simulink model "hyd_hyb_2_int_cont_Final"  (Simulink 8.2)
settings: Solver=ode4  StartTime=0  StopTime=3005  FixedStep=0.01  MaxStep=.4  RelTol=1e-8
InitFcn:
  | const_3_new
values from neighbouring files (symbols this model uses):
  Af = 6.3    [brk_enrg.m]    (also in brk_enrg_1.m)
  BSFC_906_205 = [3.5684 4.3466 5.1668 6.0769 6.988 7.8992 8.8104 9.7336 10.8548 11.9809 13.1112 14.2571 ... (663 elements, 39x17)]    [BSFC_map_906_205.mat]
  Cd = 0.55    [brk_enrg.m]    (also in brk_enrg_1.m)
  den = 1.202    [brk_enrg.m]    (also in brk_enrg_1.m)
  fr = 0.01    [brk_enrg.m]    (also in brk_enrg_1.m)
undefined symbols (not defined in the file or in its folder): clutchRise, down_spd_2, down_spd_3, down_spd_4, down_spd_c, Driving_Cycle, fuel_density, gearshift, I_wheel, Idle_spd_eng_906, M1_hydr, p_v_15, pmax_125, qv_125, Rw, sec_eng_sfc_map, T0, T1, T_max_906, T_min, TC_spd_ratio_max, teta_new_10, torque_convertor, Twait, up_spd_1, up_spd_2, up_spd_3, up_spd_c, v_p_10, v_p_15, v_p_5
libraries: neural x1742, fl_lib x43, nesl_utility x30, sdl_lib x14, simulink x4, simulink_need_slupdate x1
(part 4 of 26)

== system hyd_hyb_2_int_cont_Final/controller1/optimized controller/SOC under 0.5/col_e_f/net_col_e_f_2_4/Layer 1 ==
  "p{1}" : Inport  PortDimensions=2
  Delays 1 : Subsystem
  "IW{1,1}" : Subsystem
  "b{1}" : Constant  Value=[3.1870017165883615;1.5888517108202425;-0.37804805527583374;-1.1180149001441948;-3.2150121471194906]
  netsum : Sum  Inputs=2  SaturateOnIntegerOverflow=on  InputSameDT=on  OutDataTypeStr=Inherit: Same as first input
  tansig : neural/Transfer Functions/tansig
  "a{1}" : Outport  InitialOutput=[0;0;0;0;0]
  wires:
  "p{1}"/1 -> Delays 1/1("p{1}")
  Delays 1/1("pd{1,1}") -> "IW{1,1}"/1("pd{1,1}")
  "IW{1,1}"/1("iz{1,1}") -> netsum/1
  "b{1}"/1 -> netsum/2
  netsum/1 -> tansig/1
  tansig/1 -> "a{1}"/1

== system hyd_hyb_2_int_cont_Final/controller1/optimized controller/SOC under 0.5/col_e_f/net_col_e_f_2_4/Layer 2 ==
  "a{1} " : Inport  PortDimensions=5
  Delays 1 : Subsystem
  "LW{2,1}" : Subsystem
  "b{2}" : Constant  Value=[-2.1782011876605245;2.0554076448718699;1.2298603286219902;-0.89936716113614468;-0.28721557149157961;-0.24676230996003104;-0.6440977364861179;-1.2306338127509255;1.7211311759643211;-2.0651300272875792]
  netsum : Sum  Inputs=2  SaturateOnIntegerOverflow=on  InputSameDT=on  OutDataTypeStr=Inherit: Same as first input
  tansig : neural/Transfer Functions/tansig
  "a{2}" : Outport  InitialOutput=[0;0;0;0;0;0;0;0;0;0]
  wires:
  "a{1} "/1 -> Delays 1/1("p{2}")
  Delays 1/1("pd{2,1}") -> "LW{2,1}"/1("ad{2,1}")
  "LW{2,1}"/1("lz{2,1}") -> netsum/1
  "b{2}"/1 -> netsum/2
  netsum/1 -> tansig/1
  tansig/1 -> "a{2}"/1

== system hyd_hyb_2_int_cont_Final/controller1/optimized controller/SOC under 0.5/col_e_f/net_col_e_f_2_4/Layer 3 ==
  "a{2} " : Inport  PortDimensions=10
  Delays 1 : Subsystem
  "LW{3,2}" : Subsystem
  "b{3}" : Constant  Value=0.88069891967558567
  netsum : Sum  Inputs=2  SaturateOnIntegerOverflow=on  InputSameDT=on  OutDataTypeStr=Inherit: Same as first input
  purelin : neural/Transfer Functions/purelin
  "a{3}" : Outport  InitialOutput=0
  wires:
  "a{2} "/1 -> Delays 1/1("p{3}")
  Delays 1/1("pd{3,2}") -> "LW{3,2}"/1("ad{3,2}")
  "LW{3,2}"/1("lz{3,2}") -> netsum/1
  "b{3}"/1 -> netsum/2
  netsum/1 -> purelin/1
  purelin/1 -> "a{3}"/1

== system hyd_hyb_2_int_cont_Final/controller1/optimized controller/SOC under 0.5/col_e_f/net_col_e_f_2_4/Process Input 1 ==
  x : Inport  PortDimensions=2
  fixunknowns : neural/Processing Functions/fixunknowns  inputSize=2  indices=[1 2]
  mapminmax : neural/Processing Functions/mapminmax  xmin=[0.0064010483261946602;0.40225]  xmax=[1.009090909090909;0.527752]  ymin=-1  ymax=1
  removeconstantrows : neural/Processing Functions/removeconstantrows  inputSize=2  keep=[1 2]
  p : Outport  PortDimensions=2
  wires:
  x/1 -> fixunknowns/1
  fixunknowns/1 -> removeconstantrows/1
  removeconstantrows/1 -> mapminmax/1
  mapminmax/1 -> p/1

== system hyd_hyb_2_int_cont_Final/controller1/optimized controller/SOC under 0.5/col_e_f/net_col_e_f_2_4/Process Output 1 ==
  a : Inport  PortDimensions=1
  mapminmax_reverse : neural/Processing Functions/mapminmax_reverse  xmin=0  xmax=0.96424337740449761  ymin=-1  ymax=1
  removeconstantrows_reverse : neural/Processing Functions/removeconstantrows_reverse  inputSize=1  constants=zeros(0,1)  rearrange=1
  y : Outport  PortDimensions=1
  wires:
  a/1 -> mapminmax_reverse/1
  mapminmax_reverse/1 -> removeconstantrows_reverse/1
  removeconstantrows_reverse/1 -> y/1

== system hyd_hyb_2_int_cont_Final/controller1/optimized controller/SOC under 0.5/col_e_f/net_col_e_f_4_5/Layer 1 ==
  "p{1}" : Inport  PortDimensions=2
  Delays 1 : Subsystem
  "IW{1,1}" : Subsystem
  "b{1}" : Constant  Value=[6.2806292292580581;5.6430633337179623;4.9428699040675612;-4.2619922724486017;-3.6535514778845468;2.9896328681278797;2.3029778837955286;1.6337499102133759;-0.88051813078209484;0.2793526252740125;0.50789388949179792;-1.0078514961654155;1.4630287312614616;2.3246897312524242;2.9777230797325829;-3.5795229522621734;4.2851583321352358;-4.986226223743337;-5.6313909550551342;6.2616529893046176]
  netsum : Sum  Inputs=2  SaturateOnIntegerOverflow=on  InputSameDT=on  OutDataTypeStr=Inherit: Same as first input
  tansig : neural/Transfer Functions/tansig
  "a{1}" : Outport  InitialOutput=[0;0;0;0;0;0;0;0;0;0;0;0;0;0;0;0;0;0;0;0]
  wires:
  "p{1}"/1 -> Delays 1/1("p{1}")
  Delays 1/1("pd{1,1}") -> "IW{1,1}"/1("pd{1,1}")
  "IW{1,1}"/1("iz{1,1}") -> netsum/1
  "b{1}"/1 -> netsum/2
  netsum/1 -> tansig/1
  tansig/1 -> "a{1}"/1

== system hyd_hyb_2_int_cont_Final/controller1/optimized controller/SOC under 0.5/col_e_f/net_col_e_f_4_5/Layer 2 ==
  "a{1} " : Inport  PortDimensions=20
  Delays 1 : Subsystem
  "LW{2,1}" : Subsystem
  "b{2}" : Constant  Value=[1.6889050227737452;-1.5966398366125047;-1.5114553194028437;-1.4193609656938586;-1.3563280059510718;1.2527618415722073;1.1049860773470304;1.193805294938213;1.0220627774516799;-0.89895684788464469;-0.82709085724455877;0.78466162175281673;0.63003503504393021;0.56915459741996099;-0.45812028507076141;0.39250587067480053;0.3072138621800331;-0.20098633077147457;0.049397562122670803;0.036839924743362153;-0.03660385580770284;-0.14959783393044784;0.20236800626272414;0.29924031316589073;-0.37480244151300107;0.51487980632788588;0.56519308531635493;-0.6582920010771226;0.72211111302575659;-0.82064724071454276;0.90350102117262521;-0.96842037466691033;-1.1096684688881748;1.1383114710157722;-1.2625762588771776;-1.3484015255301616;-1.5727816552062366;1.4561588594730721;-1.6262096633611691;-1.7069579131524728]
  netsum : Sum  Inputs=2  SaturateOnIntegerOverflow=on  InputSameDT=on  OutDataTypeStr=Inherit: Same as first input
  tansig : neural/Transfer Functions/tansig
  "a{2}" : Outport  InitialOutput=[0;0;0;0;0;0;0;0;0;0;0;0;0;0;0;0;0;0;0;0;0;0;0;0;0;0;0;0;0;0;0;0;0;0;0;0;0;0;0;0]
  wires:
  "a{1} "/1 -> Delays 1/1("p{2}")
  Delays 1/1("pd{2,1}") -> "LW{2,1}"/1("ad{2,1}")
  "LW{2,1}"/1("lz{2,1}") -> netsum/1
  "b{2}"/1 -> netsum/2
  netsum/1 -> tansig/1
  tansig/1 -> "a{2}"/1

== system hyd_hyb_2_int_cont_Final/controller1/optimized controller/SOC under 0.5/col_e_f/net_col_e_f_4_5/Layer 3 ==
  "a{2} " : Inport  PortDimensions=40
  Delays 1 : Subsystem
  "LW{3,2}" : Subsystem
  "b{3}" : Constant  Value=0.083693897910831885
  netsum : Sum  Inputs=2  SaturateOnIntegerOverflow=on  InputSameDT=on  OutDataTypeStr=Inherit: Same as first input
  purelin : neural/Transfer Functions/purelin
  "a{3}" : Outport  InitialOutput=0
  wires:
  "a{2} "/1 -> Delays 1/1("p{3}")
  Delays 1/1("pd{3,2}") -> "LW{3,2}"/1("ad{3,2}")
  "LW{3,2}"/1("lz{3,2}") -> netsum/1
  "b{3}"/1 -> netsum/2
  netsum/1 -> purelin/1
  purelin/1 -> "a{3}"/1

== system hyd_hyb_2_int_cont_Final/controller1/optimized controller/SOC under 0.5/col_e_f/net_col_e_f_4_5/Process Input 1 ==
  x : Inport  PortDimensions=2
  fixunknowns : neural/Processing Functions/fixunknowns  inputSize=2  indices=[1 2]
  mapminmax : neural/Processing Functions/mapminmax  xmin=[0.012323778098949922;0.30892799999999998]  xmax=[1.009090909090909;0.60337499999999999]  ymin=-1  ymax=1
  removeconstantrows : neural/Processing Functions/removeconstantrows  inputSize=2  keep=[1 2]
  p : Outport  PortDimensions=2
  wires:
  x/1 -> fixunknowns/1
  fixunknowns/1 -> removeconstantrows/1
  removeconstantrows/1 -> mapminmax/1
  mapminmax/1 -> p/1

== system hyd_hyb_2_int_cont_Final/controller1/optimized controller/SOC under 0.5/col_e_f/net_col_e_f_4_5/Process Output 1 ==
  a : Inport  PortDimensions=1
  mapminmax_reverse : neural/Processing Functions/mapminmax_reverse  xmin=0  xmax=1  ymin=-1  ymax=1
  removeconstantrows_reverse : neural/Processing Functions/removeconstantrows_reverse  inputSize=1  constants=zeros(0,1)  rearrange=1
  y : Outport  PortDimensions=1
  wires:
  a/1 -> mapminmax_reverse/1
  mapminmax_reverse/1 -> removeconstantrows_reverse/1
  removeconstantrows_reverse/1 -> y/1

== system hyd_hyb_2_int_cont_Final/controller1/optimized controller/SOC under 0.5/net_loc_rod_2_5/Layer 1/Delays 1 ==
  "p{1}" : Inport  PortDimensions=2
  mux : Mux  Inputs=1
  "pd{1,1}" : Outport
  wires:
  "p{1}"/1 -> mux/1
  mux/1 -> "pd{1,1}"/1

== system hyd_hyb_2_int_cont_Final/controller1/optimized controller/SOC under 0.5/net_loc_rod_2_5/Layer 1/IW{1,1} ==
  "pd{1,1}" : Inport  PortDimensions=2
  "IW{1,1}(1,:)'" : Constant  Value=[2.8371454287486109;3.3980548497776453]
  "IW{1,1}(10,:)'" : Constant  Value=[-3.7320715278377063;2.3945733603075356]
  "IW{1,1}(2,:)'" : Constant  Value=[-0.38620599400705369;-4.3996835667303289]
  "IW{1,1}(3,:)'" : Constant  Value=[-3.8051772262554069;-2.2886504265709346]
  "IW{1,1}(4,:)'" : Constant  Value=[-1.5688268882272742;-4.1530598702047925]
  "IW{1,1}(5,:)'" : Constant  Value=[3.6226038294479648;2.5499616841538226]
  "IW{1,1}(6,:)'" : Constant  Value=[-3.8056419279721339;2.2605789979564013]
  "IW{1,1}(7,:)'" : Constant  Value=[4.3429514910050218;0.80174783396663385]
  "IW{1,1}(8,:)'" : Constant  Value=[-4.2363340139509029;-1.2415231044089763]
  "IW{1,1}(9,:)'" : Constant  Value=[4.1396135028112235;1.4807503949889782]
  Mux : Mux  Inputs=10
  dotprod{1..10} (10 alike) : neural/Weight Functions/dotprod
  "iz{1,1}" : Outport
  wires:
  "IW{1,1}(1,:)'"/1 -> dotprod1/1
  "pd{1,1}"/1 -> dotprod1/2, dotprod2/2, dotprod3/2, dotprod4/2, dotprod5/2, dotprod6/2, dotprod7/2, dotprod8/2, dotprod9/2, dotprod10/2
  dotprod1/1 -> Mux/1
  "IW{1,1}(2,:)'"/1 -> dotprod2/1
  dotprod2/1 -> Mux/2
  "IW{1,1}(3,:)'"/1 -> dotprod3/1
  dotprod3/1 -> Mux/3
  "IW{1,1}(4,:)'"/1 -> dotprod4/1
  dotprod4/1 -> Mux/4
  "IW{1,1}(5,:)'"/1 -> dotprod5/1
  dotprod5/1 -> Mux/5
  "IW{1,1}(6,:)'"/1 -> dotprod6/1
  dotprod6/1 -> Mux/6
  "IW{1,1}(7,:)'"/1 -> dotprod7/1
  dotprod7/1 -> Mux/7
  "IW{1,1}(8,:)'"/1 -> dotprod8/1
  dotprod8/1 -> Mux/8
  "IW{1,1}(9,:)'"/1 -> dotprod9/1
  dotprod9/1 -> Mux/9
  "IW{1,1}(10,:)'"/1 -> dotprod10/1
  dotprod10/1 -> Mux/10
  Mux/1 -> "iz{1,1}"/1

== system hyd_hyb_2_int_cont_Final/controller1/optimized controller/SOC under 0.5/net_loc_rod_2_5/Layer 2/Delays 1 ==
  "p{2}" : Inport  PortDimensions=10
  mux : Mux  Inputs=1
  "pd{2,1}" : Outport
  wires:
  "p{2}"/1 -> mux/1
  mux/1 -> "pd{2,1}"/1

== system hyd_hyb_2_int_cont_Final/controller1/optimized controller/SOC under 0.5/net_loc_rod_2_5/Layer 2/LW{2,1} ==
  "ad{2,1}" : Inport  PortDimensions=10
  "IW{2,1}(1,:)'" : Constant  Value=[0.36577909394897484;0.7188442746173328;0.30962133173311202;0.90774383968137706;-0.72047322941943104;-0.35763504337040514;0.94295978332052777;0.51167972964850672;0.13283908153078344;-0.009472061949016921]
  "IW{2,1}(10,:)'" : Constant  Value=[-0.15310687090241454;-1.392275543653263;-0.34823180633295209;-0.053854757984927684;0.8657405983540386;-0.37917010670264706;0.053587340432769769;-0.018673881301200405;0.41387516785803574;0.46028810235609202]
  "IW{2,1}(11,:)'" : Constant  Value=[0.31441891129198196;0.87827119161903844;-0.095310122390036445;-0.21390214945960834;-0.215972573454912;0.62338418488626823;0.75676188534824229;-0.61169212255405125;0.9785958766972217;0.32831420830533048]
  "IW{2,1}(12,:)'" : Constant  Value=[1.0179813468773384;0.37813072712075135;-0.52356288072083557;0.49191633488681025;0.62563472195593517;0.88084229870424358;0.29794863281638373;-0.0069153880119677894;0.013542795042253185;0.77201252045550361]
  "IW{2,1}(13,:)'" : Constant  Value=[-0.37581033217518989;-0.034506847092548677;0.63636386570473957;0.57639855136317053;0.48780967522541474;-0.28223256483943632;-0.81871626695173338;-0.83015294035649645;-0.03522271033372798;0.92989897036788516]
  "IW{2,1}(14,:)'" : Constant  Value=[0.34092651433897314;0.29125083811504127;0.27159207209561026;0.039863049489018788;-0.12069555085129059;-0.5964063392045702;-0.63165763204949499;-0.93972228253957557;0.63605573591932718;1.0158012588676575]
  "IW{2,1}(15,:)'" : Constant  Value=[-0.17539988660764949;0.095314696969921217;0.5882789019958069;-0.33294486648863914;-1.0454774856378681;0.62673797625323258;-0.19387930836040776;0.76061384776961294;-0.59940299527968854;0.58077422552225522]
  "IW{2,1}(2,:)'" : Constant  Value=[0.20859424245761346;0.69278916026248716;0.12840106063636841;0.94409160048510288;0.18650758244976126;-0.1045972710840137;-0.36528008838264364;0.66769241547874492;0.8880035930386162;0.83427661923850871]
  "IW{2,1}(3,:)'" : Constant  Value=[0.99819345834729811;-0.54672616513195105;0.49761816110077978;-0.69218605147105938;-0.53561333337743788;-0.51401041578293538;0.38258402514787926;0.65245101881301171;0.44211664098207165;0.16951259683061171]
  "IW{2,1}(4,:)'" : Constant  Value=[-0.59480453673955969;0.18018562460179566;0.03639212470669427;-0.87003975217507601;-1.0475566604995461;-0.59465649936940002;-0.18829839287195324;-0.35213692243947686;0.1337875372338829;0.81445844862201877]
  "IW{2,1}(5,:)'" : Constant  Value=[0.52075104259420935;0.10882883836078923;0.98267115770143898;0.37303221031414002;0.51973470938841448;0.6647823263974566;0.70331721011207382;0.070414809191739688;0.60586999238453032;0.48638566020184981]
  "IW{2,1}(6,:)'" : Constant  Value=[-0.59488004557922225;0.1076529862156044;-0.54302955402149111;-0.84458837008353282;-0.56768210858043855;-0.1057055709492931;0.52279195774453535;-0.82845571892803016;0.80896560665274808;0.21005615846354764]
  "IW{2,1}(7,:)'" : Constant  Value=[-0.64998354345013187;0.63177299599840386;-0.6727410431647276;0.043485386899027791;-0.098377437238256427;0.66215096812043084;-0.56831621949621436;-0.6624957646194225;0.83463929818704008;-0.43192190435249955]
  "IW{2,1}(8,:)'" : Constant  Value=[0.18180503029233497;-0.41913504689938086;-0.78679130178224443;0.12666872326851558;0.41799017038755315;-0.28802280988126733;0.78171786343162231;-0.78082054106035303;-0.98262402692318418;0.29908714862463193]
  "IW{2,1}(9,:)'" : Constant  Value=[-0.09736174060600955;-0.33598967647699857;-0.77339177813873405;0.64866727726236328;-0.28001211677648657;0.48478497639523926;0.89230472053981214;0.30786808250151909;0.67294154233326897;-0.77542089576711015]
  Mux : Mux  Inputs=15
  dotprod{1..15} (15 alike) : neural/Weight Functions/dotprod
  "lz{2,1}" : Outport
  wires:
  "IW{2,1}(1,:)'"/1 -> dotprod1/1
  "ad{2,1}"/1 -> dotprod1/2, dotprod2/2, dotprod3/2, dotprod4/2, dotprod5/2, dotprod6/2, dotprod7/2, dotprod8/2, dotprod9/2, dotprod10/2, dotprod11/2, dotprod12/2, dotprod13/2, dotprod14/2, dotprod15/2
  dotprod1/1 -> Mux/1
  "IW{2,1}(2,:)'"/1 -> dotprod2/1
  dotprod2/1 -> Mux/2
  "IW{2,1}(3,:)'"/1 -> dotprod3/1
  dotprod3/1 -> Mux/3
  "IW{2,1}(4,:)'"/1 -> dotprod4/1
  dotprod4/1 -> Mux/4
  "IW{2,1}(5,:)'"/1 -> dotprod5/1
  dotprod5/1 -> Mux/5
  "IW{2,1}(6,:)'"/1 -> dotprod6/1
  dotprod6/1 -> Mux/6
  "IW{2,1}(7,:)'"/1 -> dotprod7/1
  dotprod7/1 -> Mux/7
  "IW{2,1}(8,:)'"/1 -> dotprod8/1
  dotprod8/1 -> Mux/8
  "IW{2,1}(9,:)'"/1 -> dotprod9/1
  dotprod9/1 -> Mux/9
  "IW{2,1}(10,:)'"/1 -> dotprod10/1
  dotprod10/1 -> Mux/10
  "IW{2,1}(11,:)'"/1 -> dotprod11/1
  dotprod11/1 -> Mux/11
  "IW{2,1}(12,:)'"/1 -> dotprod12/1
  dotprod12/1 -> Mux/12
  "IW{2,1}(13,:)'"/1 -> dotprod13/1
  dotprod13/1 -> Mux/13
  "IW{2,1}(14,:)'"/1 -> dotprod14/1
  dotprod14/1 -> Mux/14
  "IW{2,1}(15,:)'"/1 -> dotprod15/1
  dotprod15/1 -> Mux/15
  Mux/1 -> "lz{2,1}"/1

== system hyd_hyb_2_int_cont_Final/controller1/optimized controller/SOC under 0.5/net_loc_rod_2_5/Layer 3/Delays 1 ==
  "p{3}" : Inport  PortDimensions=15
  mux : Mux  Inputs=1
  "pd{3,2}" : Outport
  wires:
  "p{3}"/1 -> mux/1
  mux/1 -> "pd{3,2}"/1

== system hyd_hyb_2_int_cont_Final/controller1/optimized controller/SOC under 0.5/net_loc_rod_2_5/Layer 3/LW{3,2} ==
  "ad{3,2}" : Inport  PortDimensions=15
  "IW{3,2}(1,:)'" : Constant  Value=[0.066883313762723828;0.85456989449721255;0.08483054346333925;-0.92489041669016614;-0.73401408045274952;0.76281822729255866;0.040247014242946022;0.67238278720191313;-0.62277763716735424;0.015480015065924889;0.32633252164383725;-0.86229386106999673;0.23595077532201253;-0.19159529926576901;-0.83594870790627607]
  Mux : Mux  Inputs=1
  dotprod1 : neural/Weight Functions/dotprod
  "lz{3,2}" : Outport
  wires:
  "IW{3,2}(1,:)'"/1 -> dotprod1/1
  "ad{3,2}"/1 -> dotprod1/2
  dotprod1/1 -> Mux/1
  Mux/1 -> "lz{3,2}"/1

== system hyd_hyb_2_int_cont_Final/controller1/optimized controller/SOC upper 0.5/SOC under 0.6/net_col_a_b_5_6/Layer 1 ==
  "p{1}" : Inport  PortDimensions=2
  Delays 1 : Subsystem
  "IW{1,1}" : Subsystem
  "b{1}" : Constant  Value=[-5.422100268614134;-4.6164759317401209;3.8856097524059399;-3.0640877202891303;2.3315261838129859;-1.5163056552755472;0.71285225094314353;0.0109599414209173;0.84047785527208274;-1.5772689364637402;-2.5694211307864583;3.1307185882574222;3.6899080156575645;-4.6423827027415951;5.4135020598044674]
  netsum : Sum  Inputs=2  SaturateOnIntegerOverflow=on  InputSameDT=on  OutDataTypeStr=Inherit: Same as first input
  tansig : neural/Transfer Functions/tansig
  "a{1}" : Outport  InitialOutput=[0;0;0;0;0;0;0;0;0;0;0;0;0;0;0]
  wires:
  "p{1}"/1 -> Delays 1/1("p{1}")
  Delays 1/1("pd{1,1}") -> "IW{1,1}"/1("pd{1,1}")
  "IW{1,1}"/1("iz{1,1}") -> netsum/1
  "b{1}"/1 -> netsum/2
  netsum/1 -> tansig/1
  tansig/1 -> "a{1}"/1

== system hyd_hyb_2_int_cont_Final/controller1/optimized controller/SOC upper 0.5/SOC under 0.6/net_col_a_b_5_6/Layer 2 ==
  "a{1} " : Inport  PortDimensions=15
  Delays 1 : Subsystem
  "LW{2,1}" : Subsystem
  "b{2}" : Constant  Value=[-1.7296561762017109;-1.2150006121965566;0.87865467441810763;0.64117562576410336;0.156481692895798;0.13968981028334582;-0.49421033637787221;0.70274264281099108;1.2505105446261093;1.6173752925472764]
  netsum : Sum  Inputs=2  SaturateOnIntegerOverflow=on  InputSameDT=on  OutDataTypeStr=Inherit: Same as first input
  tansig : neural/Transfer Functions/tansig
  "a{2}" : Outport  InitialOutput=[0;0;0;0;0;0;0;0;0;0]
  wires:
  "a{1} "/1 -> Delays 1/1("p{2}")
  Delays 1/1("pd{2,1}") -> "LW{2,1}"/1("ad{2,1}")
  "LW{2,1}"/1("lz{2,1}") -> netsum/1
  "b{2}"/1 -> netsum/2
  netsum/1 -> tansig/1
  tansig/1 -> "a{2}"/1

== system hyd_hyb_2_int_cont_Final/controller1/optimized controller/SOC upper 0.5/SOC under 0.6/net_col_a_b_5_6/Layer 3 ==
  "a{2} " : Inport  PortDimensions=10
  Delays 1 : Subsystem
  "LW{3,2}" : Subsystem
  "b{3}" : Constant  Value=-0.84063937418587731
  netsum : Sum  Inputs=2  SaturateOnIntegerOverflow=on  InputSameDT=on  OutDataTypeStr=Inherit: Same as first input
  purelin : neural/Transfer Functions/purelin
  "a{3}" : Outport  InitialOutput=0
  wires:
  "a{2} "/1 -> Delays 1/1("p{3}")
  Delays 1/1("pd{3,2}") -> "LW{3,2}"/1("ad{3,2}")
  "LW{3,2}"/1("lz{3,2}") -> netsum/1
  "b{3}"/1 -> netsum/2
  netsum/1 -> purelin/1
  purelin/1 -> "a{3}"/1

== system hyd_hyb_2_int_cont_Final/controller1/optimized controller/SOC upper 0.5/SOC under 0.6/net_col_a_b_5_6/Process Input 1 ==
  x : Inport  PortDimensions=2
  fixunknowns : neural/Processing Functions/fixunknowns  inputSize=2  indices=[1 2]
  mapminmax : neural/Processing Functions/mapminmax  xmin=[0.012971772427115386;0.46553733333333297]  xmax=[1;0.93965599999999994]  ymin=-1  ymax=1
  removeconstantrows : neural/Processing Functions/removeconstantrows  inputSize=2  keep=[1 2]
  p : Outport  PortDimensions=2
  wires:
  x/1 -> fixunknowns/1
  fixunknowns/1 -> removeconstantrows/1
  removeconstantrows/1 -> mapminmax/1
  mapminmax/1 -> p/1

== system hyd_hyb_2_int_cont_Final/controller1/optimized controller/SOC upper 0.5/SOC under 0.6/net_col_a_b_5_6/Process Output 1 ==
  a : Inport  PortDimensions=1
  mapminmax_reverse : neural/Processing Functions/mapminmax_reverse  xmin=0  xmax=1  ymin=-1  ymax=1
  removeconstantrows_reverse : neural/Processing Functions/removeconstantrows_reverse  inputSize=1  constants=zeros(0,1)  rearrange=1
  y : Outport  PortDimensions=1
  wires:
  a/1 -> mapminmax_reverse/1
  mapminmax_reverse/1 -> removeconstantrows_reverse/1
  removeconstantrows_reverse/1 -> y/1

== system hyd_hyb_2_int_cont_Final/controller1/optimized controller/SOC upper 0.5/SOC under 0.6/net_col_c_d_5_6/Layer 1 ==
  "p{1}" : Inport  PortDimensions=2
  Delays 1 : Subsystem
  "IW{1,1}" : Subsystem
  "b{1}" : Constant  Value=[-8.2825171004852969;-7.7884979565050276;7.3059703876936615;6.8263811255739286;6.3224546773535968;5.8380011537939929;-5.3591275616748728;-4.9619649612627033;-4.3855649268551335;-3.9040079691843612;3.4330320115235744;-2.9428333814550571;2.4336099681126804;-1.9235743654967514;-1.4584194975099747;-0.99318705748051372;-0.48139259908746823;0.016718629989637572;0.47600780483803373;-0.97888106178895162;-1.4630862071434483;1.9891000196516031;-2.6325960903318304;2.9353673705026169;-3.3901678617903399;3.9034393026749621;4.3715541612814279;-4.8652600943342197;-5.3622766242886826;-5.8323177606435213;6.4279475503741299;-6.8365979078274384;7.3738234590691603;7.7947986836768495;8.29597045879418]
  netsum : Sum  Inputs=2  SaturateOnIntegerOverflow=on  InputSameDT=on  OutDataTypeStr=Inherit: Same as first input
  tansig : neural/Transfer Functions/tansig
  "a{1}" : Outport  InitialOutput=[0;0;0;0;0;0;0;0;0;0;0;0;0;0;0;0;0;0;0;0;0;0;0;0;0;0;0;0;0;0;0;0;0;0;0]
  wires:
  "p{1}"/1 -> Delays 1/1("p{1}")
  Delays 1/1("pd{1,1}") -> "IW{1,1}"/1("pd{1,1}")
  "IW{1,1}"/1("iz{1,1}") -> netsum/1
  "b{1}"/1 -> netsum/2
  netsum/1 -> tansig/1
  tansig/1 -> "a{1}"/1

== system hyd_hyb_2_int_cont_Final/controller1/optimized controller/SOC upper 0.5/SOC under 0.6/net_col_c_d_5_6/Layer 2 ==
  "a{1} " : Inport  PortDimensions=35
  Delays 1 : Subsystem
  "LW{2,1}" : Subsystem
  "b{2}" : Constant  Value=[-1.536026974143933;1.4440490486439927;1.4116674797092896;1.3827521368296065;-1.2773302574633454;-1.2053915770045356;-1.1151655845540496;-1.0708349015730294;0.98042316538591645;0.92400185380557087;0.85309247717256687;0.76871419232437599;-0.70863566789403398;-0.64980834222296413;-0.59234963746251257;-0.50011229546283387;-0.43243037178816179;0.3775921411699466;-0.28331248324855512;-0.21871779280325679;-0.16404438767874033;-0.10474172799066278;0.0071076031033370192;0.088234481404411647;-0.12806284506645185;-0.1993744853444972;0.26305267290643747;0.35964674414275016;-0.42338227463453476;-0.52895269787297239;-0.59160570320256067;-0.64237640639733551;-0.70743270625135846;0.78067936189899567;-0.85633781523854058;-0.91788792336078784;-0.93739362962596495;1.0298599780086737;-1.1759477369169622;-1.2032446252230675;-1.2773721412372829;-1.3432047410267649;-1.4365739378820808;-1.5073201621454941;1.5628709490569166]
  netsum : Sum  Inputs=2  SaturateOnIntegerOverflow=on  InputSameDT=on  OutDataTypeStr=Inherit: Same as first input
  tansig : neural/Transfer Functions/tansig
  "a{2}" : Outport  InitialOutput=[0;0;0;0;0;0;0;0;0;0;0;0;0;0;0;0;0;0;0;0;0;0;0;0;0;0;0;0;0;0;0;0;0;0;0;0;0;0;0;0;0;0;0;0;0]
  wires:
  "a{1} "/1 -> Delays 1/1("p{2}")
  Delays 1/1("pd{2,1}") -> "LW{2,1}"/1("ad{2,1}")
  "LW{2,1}"/1("lz{2,1}") -> netsum/1
  "b{2}"/1 -> netsum/2
  netsum/1 -> tansig/1
  tansig/1 -> "a{2}"/1

== system hyd_hyb_2_int_cont_Final/controller1/optimized controller/SOC upper 0.5/SOC under 0.6/net_col_c_d_5_6/Layer 3 ==
  "a{2} " : Inport  PortDimensions=45
  Delays 1 : Subsystem
  "LW{3,2}" : Subsystem
  "b{3}" : Constant  Value=0.23481179512745601
  netsum : Sum  Inputs=2  SaturateOnIntegerOverflow=on  InputSameDT=on  OutDataTypeStr=Inherit: Same as first input
  purelin : neural/Transfer Functions/purelin
  "a{3}" : Outport  InitialOutput=0
  wires:
  "a{2} "/1 -> Delays 1/1("p{3}")
  Delays 1/1("pd{3,2}") -> "LW{3,2}"/1("ad{3,2}")
  "LW{3,2}"/1("lz{3,2}") -> netsum/1
  "b{3}"/1 -> netsum/2
  netsum/1 -> purelin/1
  purelin/1 -> "a{3}"/1

== system hyd_hyb_2_int_cont_Final/controller1/optimized controller/SOC upper 0.5/SOC under 0.6/net_col_c_d_5_6/Process Input 1 ==
  x : Inport  PortDimensions=2
  fixunknowns : neural/Processing Functions/fixunknowns  inputSize=2  indices=[1 2]
  mapminmax : neural/Processing Functions/mapminmax  xmin=[0.072950728864878897;0.36846099999999998]  xmax=[1;0.728877]  ymin=-1  ymax=1
  removeconstantrows : neural/Processing Functions/removeconstantrows  inputSize=2  keep=[1 2]
  p : Outport  PortDimensions=2
  wires:
  x/1 -> fixunknowns/1
  fixunknowns/1 -> removeconstantrows/1
  removeconstantrows/1 -> mapminmax/1
  mapminmax/1 -> p/1

== system hyd_hyb_2_int_cont_Final/controller1/optimized controller/SOC upper 0.5/SOC under 0.6/net_col_c_d_5_6/Process Output 1 ==
  a : Inport  PortDimensions=1
  mapminmax_reverse : neural/Processing Functions/mapminmax_reverse  xmin=0  xmax=1  ymin=-1  ymax=1
  removeconstantrows_reverse : neural/Processing Functions/removeconstantrows_reverse  inputSize=1  constants=zeros(0,1)  rearrange=1
  y : Outport  PortDimensions=1
  wires:
  a/1 -> mapminmax_reverse/1
  mapminmax_reverse/1 -> removeconstantrows_reverse/1
  removeconstantrows_reverse/1 -> y/1

== system hyd_hyb_2_int_cont_Final/controller1/optimized controller/SOC upper 0.5/SOC under 0.6/net_col_e_f_5_6/Layer 1 ==
  "p{1}" : Inport  PortDimensions=2
  Delays 1 : Subsystem
  "IW{1,1}" : Subsystem
  "b{1}" : Constant  Value=[7.6687154310116963;7.1265103205122102;-6.6298380060245217;-6.0710604362125311;5.5667220672055802;5.0065812960130085;4.4902349690071324;-3.9440940284275396;-3.432056942606073;2.9091254282025707;2.3792886190778688;-1.8008309082200111;1.3483753230368505;-0.75551460119655001;0.27384691484288776;0.27490521650320932;-0.78185759892251983;1.4089660121965983;-1.8210218879419833;-2.3860980972179702;-2.8074115054280151;3.4438800733701034;-3.9386908557878653;4.4609611630668775;-4.9953186339802986;-5.6208762628540123;6.0829715971602232;-6.6226610429497104;-7.15788867047696;-7.6741378399211202]
  netsum : Sum  Inputs=2  SaturateOnIntegerOverflow=on  InputSameDT=on  OutDataTypeStr=Inherit: Same as first input
  tansig : neural/Transfer Functions/tansig
  "a{1}" : Outport  InitialOutput=[0;0;0;0;0;0;0;0;0;0;0;0;0;0;0;0;0;0;0;0;0;0;0;0;0;0;0;0;0;0]
  wires:
  "p{1}"/1 -> Delays 1/1("p{1}")
  Delays 1/1("pd{1,1}") -> "IW{1,1}"/1("pd{1,1}")
  "IW{1,1}"/1("iz{1,1}") -> netsum/1
  "b{1}"/1 -> netsum/2
  netsum/1 -> tansig/1
  tansig/1 -> "a{1}"/1

== system hyd_hyb_2_int_cont_Final/controller1/optimized controller/SOC upper 0.5/SOC under 0.6/net_col_e_f_5_6/Layer 2 ==
  "a{1} " : Inport  PortDimensions=30
  Delays 1 : Subsystem
  "LW{2,1}" : Subsystem
  "b{2}" : Constant  Value=[1.508210566636943;1.1870500208099775;-0.85276762197885692;-0.40857991453644638;0.17621325952997052;-0.22893289067192346;0.57057224723412125;0.81008100008085504;1.1334859864015414;-1.4944903950594615]
  netsum : Sum  Inputs=2  SaturateOnIntegerOverflow=on  InputSameDT=on  OutDataTypeStr=Inherit: Same as first input
  tansig : neural/Transfer Functions/tansig
  "a{2}" : Outport  InitialOutput=[0;0;0;0;0;0;0;0;0;0]
  wires:
  "a{1} "/1 -> Delays 1/1("p{2}")
  Delays 1/1("pd{2,1}") -> "LW{2,1}"/1("ad{2,1}")
  "LW{2,1}"/1("lz{2,1}") -> netsum/1
  "b{2}"/1 -> netsum/2
  netsum/1 -> tansig/1
  tansig/1 -> "a{2}"/1

== system hyd_hyb_2_int_cont_Final/controller1/optimized controller/SOC upper 0.5/SOC under 0.6/net_col_e_f_5_6/Layer 3 ==
  "a{2} " : Inport  PortDimensions=10
  Delays 1 : Subsystem
  "LW{3,2}" : Subsystem
  "b{3}" : Constant  Value=0.46097967404061674
  netsum : Sum  Inputs=2  SaturateOnIntegerOverflow=on  InputSameDT=on  OutDataTypeStr=Inherit: Same as first input
  purelin : neural/Transfer Functions/purelin
  "a{3}" : Outport  InitialOutput=0
  wires:
  "a{2} "/1 -> Delays 1/1("p{3}")
  Delays 1/1("pd{3,2}") -> "LW{3,2}"/1("ad{3,2}")
  "LW{3,2}"/1("lz{3,2}") -> netsum/1
  "b{3}"/1 -> netsum/2
  netsum/1 -> purelin/1
  purelin/1 -> "a{3}"/1

== system hyd_hyb_2_int_cont_Final/controller1/optimized controller/SOC upper 0.5/SOC under 0.6/net_col_e_f_5_6/Process Input 1 ==
  x : Inport  PortDimensions=2
  fixunknowns : neural/Processing Functions/fixunknowns  inputSize=2  indices=[1 2]
  mapminmax : neural/Processing Functions/mapminmax  xmin=[0.033281760391524917;0.22204199999999999]  xmax=[1.009090909090909;0.58245800000000003]  ymin=-1  ymax=1
  removeconstantrows : neural/Processing Functions/removeconstantrows  inputSize=2  keep=[1 2]
  p : Outport  PortDimensions=2
  wires:
  x/1 -> fixunknowns/1
  fixunknowns/1 -> removeconstantrows/1
  removeconstantrows/1 -> mapminmax/1
  mapminmax/1 -> p/1

== system hyd_hyb_2_int_cont_Final/controller1/optimized controller/SOC upper 0.5/SOC under 0.6/net_col_e_f_5_6/Process Output 1 ==
  a : Inport  PortDimensions=1
  mapminmax_reverse : neural/Processing Functions/mapminmax_reverse  xmin=0  xmax=1  ymin=-1  ymax=1
  removeconstantrows_reverse : neural/Processing Functions/removeconstantrows_reverse  inputSize=1  constants=zeros(0,1)  rearrange=1
  y : Outport  PortDimensions=1
  wires:
  a/1 -> mapminmax_reverse/1
  mapminmax_reverse/1 -> removeconstantrows_reverse/1
  removeconstantrows_reverse/1 -> y/1

== system hyd_hyb_2_int_cont_Final/controller1/optimized controller/SOC upper 0.5/SOC under 0.6/net_loc_rod_5_6/Layer 1 ==
  "p{1}" : Inport  PortDimensions=2
  Delays 1 : Subsystem
  "IW{1,1}" : Subsystem
  "b{1}" : Constant  Value=[8.8632434682592827;-8.4024431058040552;-7.9438731625359278;-7.4913478065092471;-7.0390406700364885;-6.6430262624741756;6.1213305426626912;-5.6637210659388604;5.2246182224571935;4.7702996152681321;-4.3530551608801051;-3.8516886852906174;3.4065593448945468;2.9747770793332715;2.5084817143298634;2.0332347553611236;-1.3816197264599939;1.1245791413495636;-0.66785246258738729;0.18864558268796564;0.19935005396268374;0.64680714285405738;-1.1105248385243189;1.5647978869927768;-2.0588350347453672;-2.5473670707461511;2.957204742153912;3.4169273882961049;3.8794251841367982;-4.2990672449579277;-4.7554677796654721;5.2157446010828457;-5.6854215407425794;6.2663047453818015;-6.6011666950210577;7.0640200516703748;-7.4063677328570749;-7.9521169456896157;-8.3730482681647995;-8.8153243839095019]
  netsum : Sum  Inputs=2  SaturateOnIntegerOverflow=on  InputSameDT=on  OutDataTypeStr=Inherit: Same as first input
  tansig : neural/Transfer Functions/tansig
  "a{1}" : Outport  InitialOutput=[0;0;0;0;0;0;0;0;0;0;0;0;0;0;0;0;0;0;0;0;0;0;0;0;0;0;0;0;0;0;0;0;0;0;0;0;0;0;0;0]
  wires:
  "p{1}"/1 -> Delays 1/1("p{1}")
  Delays 1/1("pd{1,1}") -> "IW{1,1}"/1("pd{1,1}")
  "IW{1,1}"/1("iz{1,1}") -> netsum/1
  "b{1}"/1 -> netsum/2
  netsum/1 -> tansig/1
  tansig/1 -> "a{1}"/1

== system hyd_hyb_2_int_cont_Final/controller1/optimized controller/SOC upper 0.5/SOC under 0.6/net_loc_rod_5_6/Layer 2 ==
  "a{1} " : Inport  PortDimensions=40
  Delays 1 : Subsystem
  "LW{2,1}" : Subsystem
  "b{2}" : Constant  Value=[1.5536731790721021;-1.4752576275799514;1.4447431772976769;-1.4049951842949373;-1.3421250197047605;1.296784104954156;-1.2377992308367498;-1.1951363868937808;-1.1436917552533665;-1.0477873909756037;1.0399750464799453;-0.98306721343134096;-0.88252070575259389;0.86374006500674616;0.86297354381618008;-0.74151705347125418;-0.67586888960022085;0.66158620886656261;0.59522931524758671;0.55975640872396437;-0.56622409242359617;0.45938697145945695;-0.40070676881483702;0.35107234729512005;0.28564909473600081;-0.26304665938173283;0.097150141446890825;0.13168420526362354;-0.058709142813323428;-0.015001976205091028;-0.027310194017245118;-0.040753047503139517;0.17901525749116948;-0.197365100477086;0.21194185485691444;-0.27798418411899933;0.3459188479144476;0.40152331187541546;0.47087620147883885;0.49013879086259432;-0.54849603931418811;-0.55530513248979718;-0.64915168300786263;0.70999620039365652;0.69211163977415169;-0.85282580049544532;-0.88236075114587753;-0.92615481600950578;-0.97162167673148259;-1.0243951955115351;-1.0656365652523343;1.0859186235302416;-1.1899278852548585;-1.2149721420985302;1.2763725501762624;1.3302348955764529;-1.3925813317999192;-1.4441242230464266;1.5006538115527455;-1.5256039014677996]
  netsum : Sum  Inputs=2  SaturateOnIntegerOverflow=on  InputSameDT=on  OutDataTypeStr=Inherit: Same as first input
  tansig : neural/Transfer Functions/tansig
  "a{2}" : Outport  InitialOutput=[0;0;0;0;0;0;0;0;0;0;0;0;0;0;0;0;0;0;0;0;0;0;0;0;0;0;0;0;0;0;0;0;0;0;0;0;0;0;0;0;0;0;0;0;0;0;0;0;0;0;0;0;0;0;0;0;0;0;0;0]
  wires:
  "a{1} "/1 -> Delays 1/1("p{2}")
  Delays 1/1("pd{2,1}") -> "LW{2,1}"/1("ad{2,1}")
  "LW{2,1}"/1("lz{2,1}") -> netsum/1
  "b{2}"/1 -> netsum/2
  netsum/1 -> tansig/1
  tansig/1 -> "a{2}"/1

== system hyd_hyb_2_int_cont_Final/controller1/optimized controller/SOC upper 0.5/SOC under 0.6/net_loc_rod_5_6/Layer 3 ==
  "a{2} " : Inport  PortDimensions=60
  Delays 1 : Subsystem
  "LW{3,2}" : Subsystem
  "b{3}" : Constant  Value=-0.74715472770271352
  netsum : Sum  Inputs=2  SaturateOnIntegerOverflow=on  InputSameDT=on  OutDataTypeStr=Inherit: Same as first input
  purelin : neural/Transfer Functions/purelin
  "a{3}" : Outport  InitialOutput=0
  wires:
  "a{2} "/1 -> Delays 1/1("p{3}")
  Delays 1/1("pd{3,2}") -> "LW{3,2}"/1("ad{3,2}")
  "LW{3,2}"/1("lz{3,2}") -> netsum/1
  "b{3}"/1 -> netsum/2
  netsum/1 -> purelin/1
  purelin/1 -> "a{3}"/1

== system hyd_hyb_2_int_cont_Final/controller1/optimized controller/SOC upper 0.5/SOC under 0.6/net_loc_rod_5_6/Process Input 1 ==
  x : Inport  PortDimensions=2
  fixunknowns : neural/Processing Functions/fixunknowns  inputSize=2  indices=[1 2]
  mapminmax : neural/Processing Functions/mapminmax  xmin=[0.020662111268763654;0.24778600000000001]  xmax=[1;0.61624699999999999]  ymin=-1  ymax=1
  removeconstantrows : neural/Processing Functions/removeconstantrows  inputSize=2  keep=[1 2]
  p : Outport  PortDimensions=2
  wires:
  x/1 -> fixunknowns/1
  fixunknowns/1 -> removeconstantrows/1
  removeconstantrows/1 -> mapminmax/1
  mapminmax/1 -> p/1

== system hyd_hyb_2_int_cont_Final/controller1/optimized controller/SOC upper 0.5/SOC under 0.6/net_loc_rod_5_6/Process Output 1 ==
  a : Inport  PortDimensions=1
  mapminmax_reverse : neural/Processing Functions/mapminmax_reverse  xmin=0  xmax=1  ymin=-1  ymax=1
  removeconstantrows_reverse : neural/Processing Functions/removeconstantrows_reverse  inputSize=1  constants=zeros(0,1)  rearrange=1
  y : Outport  PortDimensions=1
  wires:
  a/1 -> mapminmax_reverse/1
  mapminmax_reverse/1 -> removeconstantrows_reverse/1
  removeconstantrows_reverse/1 -> y/1

== system hyd_hyb_2_int_cont_Final/controller1/optimized controller/SOC upper 0.5/SOC upper 0.6/SOC under 0.7/net_col_a_b_6_1 ==
  Input : Inport  PortDimensions=2
  Layer 1 : Subsystem
  Layer 2 : Subsystem
  Layer 3 : Subsystem
  Process Input 1 : Subsystem
  Process Output 1 : Subsystem
  Output : Outport  InitialOutput=0
  wires:
  Input/1 -> Process Input 1/1(x)
  Process Output 1/1(y) -> Output/1
  Process Input 1/1(p) -> Layer 1/1("p{1}")
  Layer 1/1("a{1}") -> [feedback1]
  [feedback1] -> Layer 2/1("a{1} ")
  Layer 2/1("a{2}") -> [feedback2]
  [feedback2] -> Layer 3/1("a{2} ")
  Layer 3/1("a{3}") -> Process Output 1/1(a)

== system hyd_hyb_2_int_cont_Final/controller1/optimized controller/SOC upper 0.5/SOC upper 0.6/SOC under 0.7/net_col_a_b_6_7 ==
  Input : Inport  PortDimensions=2
  Layer 1 : Subsystem
  Layer 2 : Subsystem
  Layer 3 : Subsystem
  Process Input 1 : Subsystem
  Process Output 1 : Subsystem
  Output : Outport  InitialOutput=0
  wires:
  Layer 3/1("a{3}") -> Process Output 1/1(a)
  [feedback2] -> Layer 3/1("a{2} ")
  Layer 2/1("a{2}") -> [feedback2]
  [feedback1] -> Layer 2/1("a{1} ")
  Layer 1/1("a{1}") -> [feedback1]
  Process Input 1/1(p) -> Layer 1/1("p{1}")
  Process Output 1/1(y) -> Output/1
  Input/1 -> Process Input 1/1(x)

== system hyd_hyb_2_int_cont_Final/controller1/optimized controller/SOC upper 0.5/SOC upper 0.6/SOC under 0.7/net_col_e_f_6_7 ==
  Input : Inport  PortDimensions=2
  Layer 1 : Subsystem
  Layer 2 : Subsystem
  Layer 3 : Subsystem
  Process Input 1 : Subsystem
  Process Output 1 : Subsystem
  Output : Outport  InitialOutput=0
  wires:
  Layer 3/1("a{3}") -> Process Output 1/1(a)
  [feedback2] -> Layer 3/1("a{2} ")
  Layer 2/1("a{2}") -> [feedback2]
  [feedback1] -> Layer 2/1("a{1} ")
  Layer 1/1("a{1}") -> [feedback1]
  Process Input 1/1(p) -> Layer 1/1("p{1}")
  Process Output 1/1(y) -> Output/1
  Input/1 -> Process Input 1/1(x)

== system hyd_hyb_2_int_cont_Final/controller1/optimized controller/SOC upper 0.5/SOC upper 0.6/SOC under 0.7/net_loc_rod_6_7 ==
  Input : Inport  PortDimensions=2
  Layer 1 : Subsystem
  Layer 2 : Subsystem
  Layer 3 : Subsystem
  Process Input 1 : Subsystem
  Process Output 1 : Subsystem
  Output : Outport  InitialOutput=0
  wires:
  Layer 3/1("a{3}") -> Process Output 1/1(a)
  [feedback2] -> Layer 3/1("a{2} ")
  Layer 2/1("a{2}") -> [feedback2]
  [feedback1] -> Layer 2/1("a{1} ")
  Layer 1/1("a{1}") -> [feedback1]
  Process Input 1/1(p) -> Layer 1/1("p{1}")
  Process Output 1/1(y) -> Output/1
  Input/1 -> Process Input 1/1(x)

== system hyd_hyb_2_int_cont_Final/controller1/optimized controller/SOC upper 0.5/SOC upper 0.6/SOC upper 0.7/SOC under 0.8 ==
  inps : Inport
  u_fuzz : Inport  Port=2
  Action Port : ActionPort  ActionType=then
  Demux : Demux
  Product{,1..3} (4 alike) : Product  RndMeth=Zero
  Saturation{1..4} (4 alike) : Saturate  UpperLimit=1  LowerLimit=0
  Sum : Sum  Inputs=++++
  net_col_a_b_7_8 : Subsystem
  net_col_c_d_7_8 : Subsystem
  net_col_e_f_7_8 : Subsystem
  net_loc_rod_7_8 : Subsystem
  T_ICE_opt : Outport
  wires:
  Sum/1 -> T_ICE_opt/1
  inps/1 -> net_loc_rod_7_8/1(Input), net_col_a_b_7_8/1(Input), net_col_c_d_7_8/1(Input), net_col_e_f_7_8/1(Input)
  net_loc_rod_7_8/1(Output) -> Saturation2/1
  Product/1 -> Sum/1
  Product1/1 -> Sum/2
  Product2/1 -> Sum/3
  Product3/1 -> Sum/4
  net_col_c_d_7_8/1(Output) -> Saturation3/1
  net_col_a_b_7_8/1(Output) -> Saturation1/1
  net_col_e_f_7_8/1(Output) -> Saturation4/1
  Saturation2/1 -> Product/1
  Saturation1/1 -> Product1/1
  Saturation3/1 -> Product2/1
  Saturation4/1 -> Product3/1
  Demux/1 -> Product1/2
  Demux/2 -> Product2/2
  Demux/3 -> Product3/2
  Demux/4 -> Product/2
  u_fuzz/1 -> Demux/1

== system hyd_hyb_2_int_cont_Final/controller1/optimized controller/SOC upper 0.5/SOC upper 0.6/SOC upper 0.7/SOC upper 0.8 ==
  inps : Inport
  u_fuzz : Inport  Port=2
  Action Port : ActionPort  ActionType=else
  Demux : Demux
  Product{,1..3} (4 alike) : Product  RndMeth=Zero
  Saturation{1..4} (4 alike) : Saturate  UpperLimit=1  LowerLimit=0
  Sum : Sum  Inputs=++++
  net_col_a_b_8_9 : Subsystem
  net_col_c_d_8_9 : Subsystem
  net_col_e_f_8_9 : Subsystem
  net_loc_rod_8_9 : Subsystem
  T_ICE_opt : Outport
  wires:
  Sum/1 -> T_ICE_opt/1
  inps/1 -> net_loc_rod_8_9/1(Input), net_col_a_b_8_9/1(Input), net_col_c_d_8_9/1(Input), net_col_e_f_8_9/1(Input)
  net_loc_rod_8_9/1(Output) -> Saturation2/1
  Product/1 -> Sum/1
  Product1/1 -> Sum/2
  Product2/1 -> Sum/3
  Product3/1 -> Sum/4
  net_col_c_d_8_9/1(Output) -> Saturation3/1
  net_col_a_b_8_9/1(Output) -> Saturation1/1
  net_col_e_f_8_9/1(Output) -> Saturation4/1
  Saturation2/1 -> Product/1
  Saturation1/1 -> Product1/1
  Saturation3/1 -> Product2/1
  Saturation4/1 -> Product3/1
  Demux/1 -> Product1/2
  Demux/2 -> Product2/2
  Demux/3 -> Product3/2
  Demux/4 -> Product/2
  u_fuzz/1 -> Demux/1

== system hyd_hyb_2_int_cont_Final/controller1/optimized controller/SOC under 0.5/col_c_d/net_col_c_d_2_4/Layer 1/Delays 1 ==
  "p{1}" : Inport  PortDimensions=2
  mux : Mux  Inputs=1
  "pd{1,1}" : Outport
  wires:
  "p{1}"/1 -> mux/1
  mux/1 -> "pd{1,1}"/1

== system hyd_hyb_2_int_cont_Final/controller1/optimized controller/SOC under 0.5/col_c_d/net_col_c_d_2_4/Layer 1/IW{1,1} ==
  "pd{1,1}" : Inport  PortDimensions=2
  "IW{1,1}(1,:)'" : Constant  Value=[6.9261746724528921;-3.2916011346245964]
  "IW{1,1}(10,:)'" : Constant  Value=[-4.9003827096974266;-5.8522914759268501]
  "IW{1,1}(11,:)'" : Constant  Value=[-4.050815770423057;-6.4667825674250548]
  "IW{1,1}(12,:)'" : Constant  Value=[6.660779621049806;-3.7985388493582732]
  "IW{1,1}(13,:)'" : Constant  Value=[7.4429981007526864;-1.8393790981813838]
  "IW{1,1}(14,:)'" : Constant  Value=[4.4246280044112059;-6.2615525979755233]
  "IW{1,1}(15,:)'" : Constant  Value=[-7.0338867792936508;3.0530247127062671]
  "IW{1,1}(16,:)'" : Constant  Value=[-0.28533609200472554;-7.6626971593412057]
  "IW{1,1}(17,:)'" : Constant  Value=[2.2111443131865638;7.3426042302534995]
  "IW{1,1}(18,:)'" : Constant  Value=[0.38878733604849114;7.6589906816417841]
  "IW{1,1}(19,:)'" : Constant  Value=[6.9083808914235787;-3.3240048620023104]
  "IW{1,1}(2,:)'" : Constant  Value=[3.2948960102653317;6.9104692520025131]
  "IW{1,1}(20,:)'" : Constant  Value=[0.94653354375634247;-7.609752438919541]
  "IW{1,1}(21,:)'" : Constant  Value=[4.6546854073657329;-6.0941282090882858]
  "IW{1,1}(22,:)'" : Constant  Value=[5.9259380018073493;4.8662925939646229]
  "IW{1,1}(23,:)'" : Constant  Value=[2.8351157744944908;-7.1249725909597244]
  "IW{1,1}(24,:)'" : Constant  Value=[-7.5918951566256201;-1.0312708310903715]
  "IW{1,1}(25,:)'" : Constant  Value=[5.4358392868731755;-5.4182289443688223]
  "IW{1,1}(26,:)'" : Constant  Value=[-4.7589600600299304;-6.0267781906018145]
  "IW{1,1}(27,:)'" : Constant  Value=[4.1917416127995235;6.411366108069668]
  "IW{1,1}(28,:)'" : Constant  Value=[-2.4152333950585239;7.2289997573298788]
  "IW{1,1}(29,:)'" : Constant  Value=[4.5454133647226795;-6.142449821054182]
  "IW{1,1}(3,:)'" : Constant  Value=[-2.4837072291086124;7.2553236889260981]
  "IW{1,1}(30,:)'" : Constant  Value=[-3.9650780518305329;-6.5662962286217113]
  "IW{1,1}(4,:)'" : Constant  Value=[7.4419722731611202;-1.8788467345997706]
  "IW{1,1}(5,:)'" : Constant  Value=[-1.4112051457237573;-7.5911646879168826]
  "IW{1,1}(6,:)'" : Constant  Value=[7.3756886862648523;2.0972469275080932]
  "IW{1,1}(7,:)'" : Constant  Value=[3.275784537007266;6.9007386886807467]
  "IW{1,1}(8,:)'" : Constant  Value=[7.1995046832004004;2.6385551878650326]
  "IW{1,1}(9,:)'" : Constant  Value=[5.0427812981617457;5.8247566308699552]
  Mux : Mux  Inputs=30
  dotprod{1..30} (30 alike) : neural/Weight Functions/dotprod
  "iz{1,1}" : Outport
  wires:
  "IW{1,1}(1,:)'"/1 -> dotprod1/1
  "pd{1,1}"/1 -> dotprod1/2, dotprod2/2, dotprod3/2, dotprod4/2, dotprod5/2, dotprod6/2, dotprod7/2, dotprod8/2, dotprod9/2, dotprod10/2, dotprod11/2, dotprod12/2, dotprod13/2, dotprod14/2, dotprod15/2, dotprod16/2, dotprod17/2, dotprod18/2, dotprod19/2, dotprod20/2, dotprod21/2, dotprod22/2, dotprod23/2, dotprod24/2, dotprod25/2, dotprod26/2, dotprod27/2, dotprod28/2, dotprod29/2, dotprod30/2
  dotprod1/1 -> Mux/1
  "IW{1,1}(2,:)'"/1 -> dotprod2/1
  dotprod2/1 -> Mux/2
  "IW{1,1}(3,:)'"/1 -> dotprod3/1
  dotprod3/1 -> Mux/3
  "IW{1,1}(4,:)'"/1 -> dotprod4/1
  dotprod4/1 -> Mux/4
  "IW{1,1}(5,:)'"/1 -> dotprod5/1
  dotprod5/1 -> Mux/5
  "IW{1,1}(6,:)'"/1 -> dotprod6/1
  dotprod6/1 -> Mux/6
  "IW{1,1}(7,:)'"/1 -> dotprod7/1
  dotprod7/1 -> Mux/7
  "IW{1,1}(8,:)'"/1 -> dotprod8/1
  dotprod8/1 -> Mux/8
  "IW{1,1}(9,:)'"/1 -> dotprod9/1
  dotprod9/1 -> Mux/9
  "IW{1,1}(10,:)'"/1 -> dotprod10/1
  dotprod10/1 -> Mux/10
  "IW{1,1}(11,:)'"/1 -> dotprod11/1
  dotprod11/1 -> Mux/11
  "IW{1,1}(12,:)'"/1 -> dotprod12/1
  dotprod12/1 -> Mux/12
  "IW{1,1}(13,:)'"/1 -> dotprod13/1
  dotprod13/1 -> Mux/13
  "IW{1,1}(14,:)'"/1 -> dotprod14/1
  dotprod14/1 -> Mux/14
  "IW{1,1}(15,:)'"/1 -> dotprod15/1
  dotprod15/1 -> Mux/15
  "IW{1,1}(16,:)'"/1 -> dotprod16/1
  dotprod16/1 -> Mux/16
  "IW{1,1}(17,:)'"/1 -> dotprod17/1
  dotprod17/1 -> Mux/17
  "IW{1,1}(18,:)'"/1 -> dotprod18/1
  dotprod18/1 -> Mux/18
  "IW{1,1}(19,:)'"/1 -> dotprod19/1
  dotprod19/1 -> Mux/19
  "IW{1,1}(20,:)'"/1 -> dotprod20/1
  dotprod20/1 -> Mux/20
  "IW{1,1}(21,:)'"/1 -> dotprod21/1
  dotprod21/1 -> Mux/21
  "IW{1,1}(22,:)'"/1 -> dotprod22/1
  dotprod22/1 -> Mux/22
  "IW{1,1}(23,:)'"/1 -> dotprod23/1
  dotprod23/1 -> Mux/23
  "IW{1,1}(24,:)'"/1 -> dotprod24/1
  dotprod24/1 -> Mux/24
  "IW{1,1}(25,:)'"/1 -> dotprod25/1
  dotprod25/1 -> Mux/25
  "IW{1,1}(26,:)'"/1 -> dotprod26/1
  dotprod26/1 -> Mux/26
  "IW{1,1}(27,:)'"/1 -> dotprod27/1
  dotprod27/1 -> Mux/27
  "IW{1,1}(28,:)'"/1 -> dotprod28/1
  dotprod28/1 -> Mux/28
  "IW{1,1}(29,:)'"/1 -> dotprod29/1
  dotprod29/1 -> Mux/29
  "IW{1,1}(30,:)'"/1 -> dotprod30/1
  dotprod30/1 -> Mux/30
  Mux/1 -> "iz{1,1}"/1

== system hyd_hyb_2_int_cont_Final/controller1/optimized controller/SOC under 0.5/col_c_d/net_col_c_d_2_4/Layer 2/Delays 1 ==
  "p{2}" : Inport  PortDimensions=30
  mux : Mux  Inputs=1
  "pd{2,1}" : Outport
  wires:
  "p{2}"/1 -> mux/1
  mux/1 -> "pd{2,1}"/1
